simulink model "Forced_SMD_System"  (R2024a)
settings: Solver=VariableStepAuto  StartTime=0.0  StopTime=5  MaxStep=0.01  RelTol=1e-3
model workspace (MAT data in the model file):
  b = 0.5
  k = 1
  m = 10
settings Model: Creator=91839
settings SolverCC: AlgebraicLoopSolver=TrustRegion
settings DataIOCC: ExternalInput=data  LoadExternalInput=on  SaveFormat=Array  DSMLogging=off  ReturnWorkspaceOutputs=off
settings DebuggingCC: UnconnectedInputMsg=warning  UnconnectedOutputMsg=warning  UnconnectedLineMsg=warning
settings ModelReferenceCC: EnableRefExpFcnMdlSchedulingChecks=on
settings SFSimCC: CustomCodeUndefinedFunction=UseInterfaceOnly
settings RTWCC: GPUComputeCapability=3.5

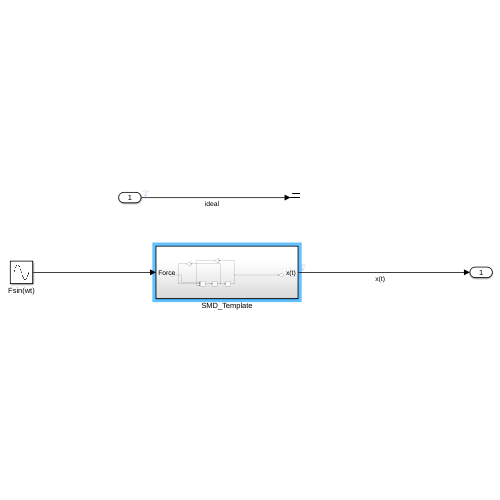
[thumbnail: Simulink's stored preview of the top-level diagram]
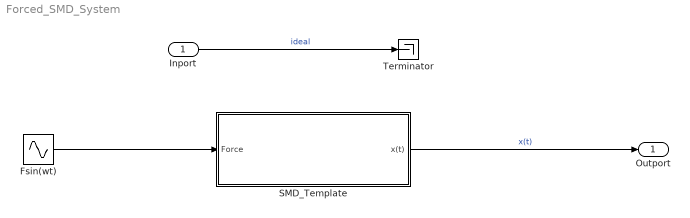
== system Forced_SMD_System ==
  Inport : Inport
  Fsin(wt) : Sin  Amplitude=100  Frequency=20  SampleTime=0
  SMD_Template : Subsystem
  Terminator : Terminator
  Outport : Outport
  wires:
  Inport/1 -> Terminator/1  "ideal"
  Fsin(wt)/1 -> SMD_Template/1(Force)
  SMD_Template/1(x(t)) -> Outport/1  "x(t)"

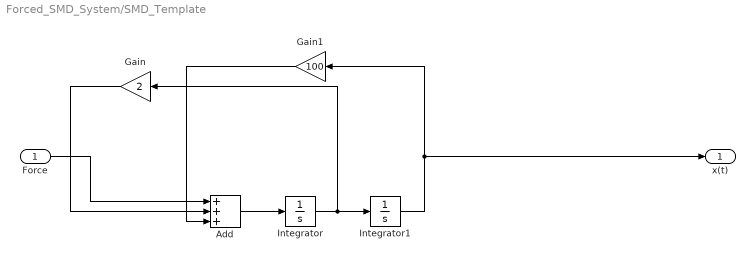
== system Forced_SMD_System/SMD_Template ==
  Force : Inport
  Add : Sum  Inputs=+++
  Gain : Gain  Gain=2
  Gain1 : Gain  Gain=100
  Integrator : Integrator  InitialCondition=0.02
  Integrator1 : Integrator
  x(t) : Outport
  wires:
  Force/1 -> Add/1
  Gain/1 -> Add/2
  Gain1/1 -> Add/3
  Add/1 -> Integrator/1
  Integrator/1 -> Gain/1, Integrator1/1
  Integrator1/1 -> x(t)/1, Gain1/1
